simulink model "syssim"  (R2016b)
settings: Solver=VariableStepAuto  StartTime=0.0  StopTime=5000.0  RelTol=1e-3
values from neighbouring files (symbols this model uses):
  Ad = sysdd.A    [trock.m]
  Bd = sysdd.B(1:2)    [trock.m]
  Cd = sysdd.C    [trock.m]
  Dd = sysdd.D(:,1:2)    [trock.m]
  Ed = sysdd.B(3:4)    [trock.m]
  Kd = sysdd.D(:,3:4)    [trock.m]
  Ts = 87.5440    (= 87.544)    [trock.m]
libraries: powerlib_meascontrol x4
settings Model: Creator=Daniel  LastModifiedBy=Daniel

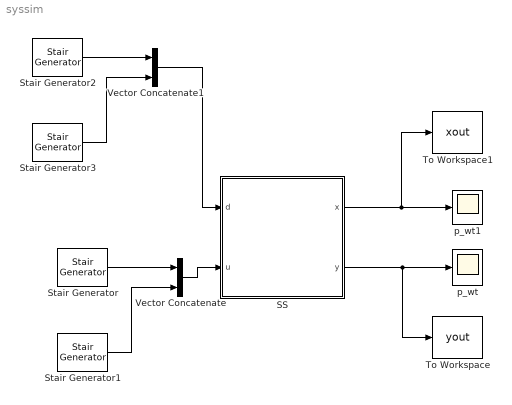
== system syssim ==
  SS : Subsystem
  Stair Generator : powerlib_meascontrol/Pulse & Signal Generators/Stair Generator  t=[0]  e=[0.5]  Ts=0.05
  Stair Generator1 : powerlib_meascontrol/Pulse & Signal Generators/Stair Generator  t=[0]  e=[0]  Ts=0.05
  Stair Generator2 : powerlib_meascontrol/Pulse & Signal Generators/Stair Generator  t=[0,3000]  e=[0,5]  Ts=0.05
  Stair Generator3 : powerlib_meascontrol/Pulse & Signal Generators/Stair Generator  t=[0,4000]  e=[0,-5]  Ts=0.05
  To Workspace : ToWorkspace  VariableName=yout  SampleTime=-1
      settings: Save2DSignal=2-D array (concatenate along first dimension)
  To Workspace1 : ToWorkspace  VariableName=xout  SampleTime=-1
      settings: Save2DSignal=2-D array (concatenate along first dimension)
  Vector Concatenate : Concatenate
  Vector Concatenate1 : Concatenate
  p_wt : Scope
  p_wt1 : Scope
  wires:
  SS/2(y) -> To Workspace/1, p_wt/1
  Stair Generator1/1 -> Vector Concatenate/2
  Stair Generator/1 -> Vector Concatenate/1
  Vector Concatenate/1 -> SS/2(u)
  Stair Generator3/1 -> Vector Concatenate1/2
  Stair Generator2/1 -> Vector Concatenate1/1
  Vector Concatenate1/1 -> SS/1(d)
  SS/1(x) -> To Workspace1/1, p_wt1/1

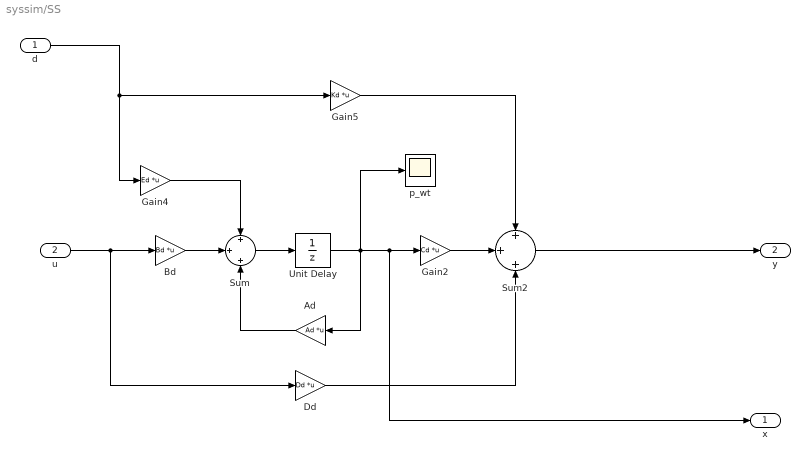
== system syssim/SS ==
  d : Inport
  u : Inport  Port=2
  Ad : Gain  Gain=Ad  Multiplication=Matrix(K*u)
      mask Display:
      | %color('cyan')
      | color('magenta')
      | disp('{\bf\fontsize{14}Ad}', 'texmode','on');
      | %disp('Ad')
  Bd : Gain  Gain=Bd  Multiplication=Matrix(K*u)
      mask Display:
      | %color('cyan')
      | color('magenta')
      | disp('{\bf\fontsize{14}Bd}', 'texmode','on');
      | %disp('Bd')
  Dd : Gain  Gain=Dd  Multiplication=Matrix(K*u)
      mask Display:
      | %color('cyan')
      | color('magenta')
      | disp('{\bf\fontsize{14}Dd}', 'texmode','on');
      | %disp('Dd')
  Gain2 : Gain  Gain=Cd  Multiplication=Matrix(K*u)
      mask Display:
      | %color('cyan')
      | color('magenta')
      | disp('{\bf\fontsize{14}Cd}', 'texmode','on');
      | %disp('Cd')
  Gain4 : Gain  Gain=Ed  Multiplication=Matrix(K*u)
      mask Display:
      | %color('cyan')
      | color('magenta')
      | disp('{\bf\fontsize{14}Ed}', 'texmode','on');
      | %disp('Ed')
  Gain5 : Gain  Gain=Kd  Multiplication=Matrix(K*u)
      mask Display:
      | %color('cyan')
      | color('magenta')
      | disp('{\bf\fontsize{14}Kd}', 'texmode','on');
      | %disp('Kd')
  Sum : Sum  Inputs=+|+|+
  Sum2 : Sum  Inputs=+|+|+
  Unit Delay : UnitDelay  InitialCondition=0.005  SampleTime=Ts
  p_wt : Scope
  x : Outport
  y : Outport  Port=2
  wires:
  Gain5/1 -> Sum2/1
  Dd/1 -> Sum2/3
  Gain2/1 -> Sum2/2
  Gain4/1 -> Sum/1
  d/1 -> Gain5/1, Gain4/1
  u/1 -> Bd/1, Dd/1
  Unit Delay/1 -> Ad/1, Gain2/1, x/1, p_wt/1
  Ad/1 -> Sum/3
  Bd/1 -> Sum/2
  Sum/1 -> Unit Delay/1
  Sum2/1 -> y/1
